simulink model "memory_test"  (Simulink 9.0)
settings: Solver=FixedStepAuto  StartTime=0.0  StopTime=10.0  FixedStep=0.1  RelTol=1e-3  EnableMultiTasking=on
settings Model: SuppressorTable=22 serialization::archive 11 0 6 0 0 0 0 0  Creator=arnaud  LastModifiedBy=hbourbou
settings DataIOCC: LimitDataPoints=on  SaveFormat=Structure  SignalLoggingSaveFormat=ModelDataLogs
settings OptimizationCC: ExpressionDepthLimit=2147483647
settings DebuggingCC: SolverPrmCheckMsg=warning  FcnCallInpInsideContextMsg=warning  StateNameClashWarn=warning  StrictBusMsg=Warning
settings GRTTargetCC: GeneratePreprocessorConditionals=Disable all  CombineOutputUpdateFcns=off  GRTInterface=on
settings ConfigComp: CovSFcnEnable=off

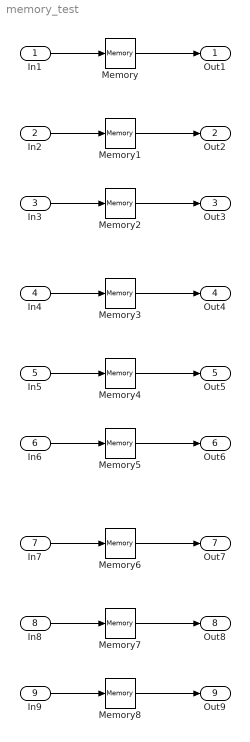
== system memory_test ==
  In1 : Inport  OutDataTypeStr=double  PortDimensions=1
  In2 : Inport  Port=2  OutDataTypeStr=double  PortDimensions=1
  In3 : Inport  Port=3  PortDimensions=1
  In4 : Inport  Port=4  OutDataTypeStr=int8  PortDimensions=1
  In5 : Inport  Port=5  OutDataTypeStr=int8  PortDimensions=1
  In6 : Inport  Port=6  OutDataTypeStr=int8  PortDimensions=1
  In7 : Inport  Port=7  OutDataTypeStr=boolean  PortDimensions=1
  In8 : Inport  Port=8  OutDataTypeStr=boolean  PortDimensions=1
  In9 : Inport  Port=9  OutDataTypeStr=boolean  PortDimensions=1
  Memory : Memory
  Memory1 : Memory  InitialCondition=0.0
  Memory2 : Memory  InitialCondition=true
  Memory3 : Memory
  Memory4 : Memory  InitialCondition=0.0
  Memory5 : Memory  InitialCondition=true
  Memory6 : Memory
  Memory7 : Memory  InitialCondition=0.0
  Memory8 : Memory  InitialCondition=true
  Out1 : Outport
  Out2 : Outport  Port=2
  Out3 : Outport  Port=3
  Out4 : Outport  Port=4
  Out5 : Outport  Port=5
  Out6 : Outport  Port=6
  Out7 : Outport  Port=7
  Out8 : Outport  Port=8
  Out9 : Outport  Port=9
  wires:
  In1/1 -> Memory/1
  Memory/1 -> Out1/1
  In2/1 -> Memory1/1
  Memory1/1 -> Out2/1
  In3/1 -> Memory2/1
  Memory2/1 -> Out3/1
  In4/1 -> Memory3/1
  Memory3/1 -> Out4/1
  In5/1 -> Memory4/1
  Memory4/1 -> Out5/1
  In6/1 -> Memory5/1
  Memory5/1 -> Out6/1
  In7/1 -> Memory6/1
  Memory6/1 -> Out7/1
  In8/1 -> Memory7/1
  Memory7/1 -> Out8/1
  In9/1 -> Memory8/1
  Memory8/1 -> Out9/1
